simulink model "CLVF"  (R2020a)
settings: Solver=FixedStepAuto  StartTime=0.0  StopTime=tsim  FixedStep=baseRate  RelTol=1e-3  EnableMultiTasking=on
values from neighbouring files (symbols this model uses):
  a = sqrt(sum(aTimesOVec.^2))    [Run_Initializer.m]
  a_max = u_max_scalar/BLACKMass    [Run_Initializer.m]
  a_prime = 0.2    [Run_Initializer.m]
  acceptableRadius = 0.05    [Run_Initializer.m]
  aTimesOVec = d + a_prime*o_hat_prime    [Run_Initializer.m]
  b = 1.0    (= 1)    [Run_Initializer.m]    (also in a_max_CLVF3D_quad.m = params(3))
  baseRate = 0.05    [Run_Initializer.m]
  BLACKInertia = model_param(4)    [Run_Initializer.m]
  BLACKMass = model_param(3)    [Run_Initializer.m]
  cntThreshold = timeThreshold/baseRate    (= 100)    [Run_Initializer.m]
  d = [0.16;0.542;0]    [Run_Initializer.m]
  drop_states_BLACK = rC_I0    [Run_Initializer.m]
  drop_states_BLUE = [ xLength/2+0.9; yLength/2+0.5; 0]    [Run_Initializer.m]
  drop_states_RED = rT_I0    [Run_Initializer.m]
  F_thrusters_BLACK = 0.25.*ones(8,1)    [Run_Initializer.m]
  F_thrusters_BLUE = 0.25.*ones(8,1)    [Run_Initializer.m]
  F_thrusters_RED = 0.25.*ones(8,1)    [Run_Initializer.m]
  finalAngle = fact*pi    (= 2.98451302091)    [Run_Initializer.m]
  home_states_BLACK = [xLength/2-0.4; yLength/2; 0]    [Run_Initializer.m]
  home_states_BLUE = [ xLength/2-0.9; yLength/2+0.5; 0]    [Run_Initializer.m]
  home_states_RED = [xLength/2+0.4; yLength/2; 0]    [Run_Initializer.m]
  init_states_BLACK = rC_I0    [Run_Initializer.m]
  init_states_BLUE = [ xLength/2+0.9; yLength/2+0.5; 0]    [Run_Initializer.m]
  init_states_RED = rT_I0    [Run_Initializer.m]
  ka = 0.01    [Run_Initializer.m]    (also in a_max_CLVF3D_quad.m = params(1))
  kc = 0.01    [Run_Initializer.m]    (also in a_max_CLVF3D_quad.m = params(2))
  kd = 5.0    (= 5)    [Run_Initializer.m]
  Kd_tb = 0.4    [Run_Initializer.m]
  Kd_tblue = 0.4    [Run_Initializer.m]
  Kd_tr = 0.4    [Run_Initializer.m]
  Kd_xb = 5    [Run_Initializer.m]
  Kd_xblue = 5    [Run_Initializer.m]
  Kd_xr = 5    [Run_Initializer.m]
  Kd_yb = 5    [Run_Initializer.m]
  Kd_yblue = 5    [Run_Initializer.m]
  Kd_yr = 5    [Run_Initializer.m]
  Kp_tb = 0.1    [Run_Initializer.m]
  Kp_tblue = 0.1    [Run_Initializer.m]
  Kp_tr = 0.1    [Run_Initializer.m]
  Kp_xb = 2    [Run_Initializer.m]
  Kp_xblue = 2    [Run_Initializer.m]
  Kp_xr = 2    [Run_Initializer.m]
  Kp_yb = 2    [Run_Initializer.m]
  Kp_yblue = 2    [Run_Initializer.m]
  Kp_yr = 2    [Run_Initializer.m]
  MPCStructure = getMPCStructure(BLACKMass, b_cone, R, Q, Q_final, u_max_scalar, kc, aTimesOVec)    [Run_Initializer.m]
  noise_variance_BLACK = 0    [Run_Initializer.m]
  noise_variance_BLUE = 0    [Run_Initializer.m]
  noise_variance_RED = 0    [Run_Initializer.m]
  o_hat_B = aTimesOVec./a    [Run_Initializer.m]
  o_hat_prime = [0;1;0]    [Run_Initializer.m]
  Phase0_End = Phase0_Duration    (= 10)    [Run_Initializer.m]
  Phase1_End = Phase0_Duration + Phase1_Duration    (= 15)    [Run_Initializer.m]
  Phase2_End = Phase0_Duration + Phase1_Duration +                                   Phase2_Duration    (= 35)    [Run_Initializer.m]
  Phase3_End = Phase0_Duration + Phase1_Duration +                                   Phase2_Duration + Phase3_Duration    [Run_Initializer.m]
  Phase3_SubPhase1_End = Phase2_End + Phase3_SubPhase1_Duration    (= 40)    [Run_Initializer.m]
  Phase3_SubPhase2_End = Phase2_End + Phase3_SubPhase1_Duration +                                   Phase3_SubPhase2_Duration    (= 45)    [Run_Initializer.m]
  Phase3_SubPhase3_End_BLACK = Phase2_End + Phase3_SubPhase1_Duration +                                   Phase3_SubPhase2_Duration +                                  Phase3_SubPhase3_Duration + Phase3_SubPhase3_and_a_half    (= 51)    [Run_Initializer.m]
  Phase3_SubPhase3_End_RED = Phase2_End + Phase3_SubPhase1_Duration +                                   Phase3_SubPhase2_Duration +                                  Phase3_SubPhase3_Duration    (= 46)    [Run_Initializer.m]
  Phase3_SubPhase4_End = Phase2_End + Phase3_SubPhase1_Duration +                                   Phase3_SubPhase2_Duration +                                  Phase3_SubPhase3_Duration +                                  Phase3_SubPhase4_Duration + Phase3_SubPhase3_and_a_half    [Run_Initializer.m]
  Phase4_End = Phase0_Duration + Phase1_Duration +                                   Phase2_Duration + Phase3_Duration +                                   Phase4_Duration    [Run_Initializer.m]
  Phase5_End = Phase0_Duration + Phase1_Duration +                                   Phase2_Duration + Phase3_Duration +                                   Phase4_Duration + Phase5_Duration    [Run_Initializer.m]
  rT_I0 = ICStructure.rT_I0{initialConditionSet}    [Run_Initializer.m]
  serverRate = 0.1    [Run_Initializer.m]
  theta_d = 30*d2r    (= 0.523598775598)    [Run_Initializer.m]    (also in a_max_LVF3D.m = rotStuff(4))
  thruster_dist2CG_BLACK = [83.42;-52.58;55.94;-60.05;54.08;-53.92;77.06;-55.94]    [Run_Initializer.m]
  thruster_dist2CG_BLUE = [83.42;-52.58;55.94;-60.05;54.08;-53.92;77.06;-55.94]    [Run_Initializer.m]
  thruster_dist2CG_RED = [49.92;-78.08;70.46;-63.54;81.08;-50.42;57.44;-75.96]    [Run_Initializer.m]
  v_max = interiorPointLVF_heur(     a_prime,      v_max,      a_max,      w_max,      rotNorm,      dockingPortNorm,      theta_d,      fact,      W_LVF,      mu,      tol,      gamma,      beta,      muFact,      muLimit )    [Run_Initializer.m]
  w_body = ICStructure.w_body{initialConditionSet}    [Run_Initializer.m]
undefined symbols (not defined in the file or in its folder): A_cone, DiscIntNeverNeededParam, FixedStep, Phase3_SubPhase3_End, platformSelection, simMode, WhoAmI
libraries: dspstat3 x18, dspsigops x11, raspberrypiBasiclib x10, embdlinuxlib x8, simulink x8, mspfiltlib x3, dsparch4 x3, dspswit3 x2, MainLibrary x2, sensehatlib x1
(part 9 of 10)

== system CLVF/Grab PhaseSpace Data via UDP/Use Hardware to Obtain States/Using RED+BLACK, or RED+BLACK+ARM/Obtain RED States/x_dot -> x2/Hold this value ==
  In1 : Inport
  Action Port : ActionPort  ActionPortLabel=if(u1 ~= 0)
  Out1 : Outport  VectorParamsAs1DForOutWhenUnconnected=off
  wires:
  In1/1 -> Out1/1

== system CLVF/Grab PhaseSpace Data via UDP/Use Hardware to Obtain States/Using RED+BLACK, or RED+BLACK+ARM/Obtain RED States/x_dot -> x3/Hold this value ==
  In1 : Inport
  Action Port : ActionPort  ActionPortLabel=if(u1 ~= 0)
  Out1 : Outport  VectorParamsAs1DForOutWhenUnconnected=off
  wires:
  In1/1 -> Out1/1

== system CLVF/Grab PhaseSpace Data via UDP/Use Hardware to Obtain States/Using RED+BLACK, or RED+BLACK+ARM/Obtain RED States/x_dot -> x4/Hold this value ==
  In1 : Inport
  Action Port : ActionPort  ActionPortLabel=if(u1 ~= 0)
  Out1 : Outport  VectorParamsAs1DForOutWhenUnconnected=off
  wires:
  In1/1 -> Out1/1

== system CLVF/Grab PhaseSpace Data via UDP/Use Hardware to Obtain States/Using RED+BLACK, or RED+BLACK+ARM/Obtain RED States/x_dot -> x5/Hold this value ==
  In1 : Inport
  Action Port : ActionPort  ActionPortLabel=if(u1 ~= 0)
  Out1 : Outport  VectorParamsAs1DForOutWhenUnconnected=off
  wires:
  In1/1 -> Out1/1

== system CLVF/Grab PhaseSpace Data via UDP/Use Hardware to Obtain States/Using RED+BLACK, or RED+BLACK+ARM/Obtain RED States/x_dot -> x6/Hold this value ==
  In1 : Inport
  Action Port : ActionPort  ActionPortLabel=if(u1 ~= 0)
  Out1 : Outport  VectorParamsAs1DForOutWhenUnconnected=off
  wires:
  In1/1 -> Out1/1

== system CLVF/Grab PhaseSpace Data via UDP/Use Hardware to Obtain States/Using RED+BLACK, or RED+BLACK+ARM/Obtain RED States/x_dot -> x7/Hold this value ==
  In1 : Inport
  Action Port : ActionPort  ActionPortLabel=if(u1 ~= 0)
  Out1 : Outport  VectorParamsAs1DForOutWhenUnconnected=off
  wires:
  In1/1 -> Out1/1

== system CLVF/Grab PhaseSpace Data via UDP/Use Hardware to Obtain States/Using RED+BLACK, or RED+BLACK+ARM/Obtain RED States/x_dot -> x8/Hold this value ==
  In1 : Inport
  Action Port : ActionPort  ActionPortLabel=if(u1 ~= 0)
  Out1 : Outport  VectorParamsAs1DForOutWhenUnconnected=off
  wires:
  In1/1 -> Out1/1

== system CLVF/Grab PhaseSpace Data via UDP/Use Hardware to Obtain States/Using RED+BLACK, or RED+BLACK+ARM/Obtain RED States/x_dot -> x9/Hold this value ==
  In1 : Inport
  Action Port : ActionPort  ActionPortLabel=if(u1 ~= 0)
  Out1 : Outport  VectorParamsAs1DForOutWhenUnconnected=off
  wires:
  In1/1 -> Out1/1

== system CLVF/Phase #3: Experiment/Change BLACK Behavior/Sub-Phase #1/Custom Discrete PD (Attitude)/x_dot -> x1/Hold this value ==
  In1 : Inport
  Action Port : ActionPort  ActionPortLabel=if(u1 ~= 0)
  Out1 : Outport  VectorParamsAs1DForOutWhenUnconnected=off
  wires:
  In1/1 -> Out1/1

== system CLVF/Phase #3: Experiment/Change BLACK Behavior/Sub-Phase #1/Custom Discrete PD (X-Position)/x_dot -> x1/Hold this value ==
  In1 : Inport
  Action Port : ActionPort  ActionPortLabel=if(u1 ~= 0)
  Out1 : Outport  VectorParamsAs1DForOutWhenUnconnected=off
  wires:
  In1/1 -> Out1/1

== system CLVF/Phase #3: Experiment/Change BLACK Behavior/Sub-Phase #1/Custom Discrete PD (Y-Position)/x_dot -> x1/Hold this value ==
  In1 : Inport
  Action Port : ActionPort  ActionPortLabel=if(u1 ~= 0)
  Out1 : Outport  VectorParamsAs1DForOutWhenUnconnected=off
  wires:
  In1/1 -> Out1/1

== system CLVF/Phase #3: Experiment/Change BLACK Behavior/Sub-Phase #4/Custom Discrete PD (Attitude)/x_dot -> x1/Hold this value ==
  In1 : Inport
  Action Port : ActionPort  ActionPortLabel=if(u1 ~= 0)
  Out1 : Outport  VectorParamsAs1DForOutWhenUnconnected=off
  wires:
  In1/1 -> Out1/1

== system CLVF/Phase #3: Experiment/Change BLACK Behavior/Sub-Phase #4/Lyapunov GNC/CLVF//LVF System/CLVF ==
  rC_I : Inport
  rT_I : Inport  Port=2
  vT_I : Inport  Port=3
  aT_I : Inport  Port=4
  CT_BI : Inport  Port=5
  wT_B : Inport  Port=6
  w_dot_B : Inport  Port=7
  vC_I : Inport  Port=8
  Action Port : ActionPort  ActionPortLabel=if(u1 == 0)
  Constant : Constant  Value=o_hat_B
  Constant1 : Constant  Value=a
  Constant2 : Constant  Value=b
  Constant3 : Constant  Value=ka
  Constant4 : Constant  Value=kc
  Derivative : Derivative
  Lyapunov Guidance + FF : MATLAB Function  TreatAsAtomicUnit=on
  Scope : Scope
  Scope1 : Scope
  Sum : Sum  Inputs=|+-
  h : Outport
  a_ff : Outport  Port=2
  wires:
  vT_I/1 -> Lyapunov Guidance + FF/3(vT_I)
  rT_I/1 -> Lyapunov Guidance + FF/2(rT_I)
  wT_B/1 -> Lyapunov Guidance + FF/6(wT_B)
  w_dot_B/1 -> Lyapunov Guidance + FF/7(w_dot_B)
  vC_I/1 -> Lyapunov Guidance + FF/8(vC_I)
  CT_BI/1 -> Lyapunov Guidance + FF/5(CT_BI)
  aT_I/1 -> Lyapunov Guidance + FF/4(aT_I)
  rC_I/1 -> Lyapunov Guidance + FF/1(rC_I)
  Lyapunov Guidance + FF/2(a_ff) -> Sum/2, Scope1/1, a_ff/1
  Lyapunov Guidance + FF/1(h) -> Derivative/1, h/1
  Derivative/1 -> Sum/1
  Sum/1 -> Scope/1
  Constant/1 -> Lyapunov Guidance + FF/9(o_hat_B)
  Constant4/1 -> Lyapunov Guidance + FF/13(kc)
  Constant2/1 -> Lyapunov Guidance + FF/11(b)
  Constant3/1 -> Lyapunov Guidance + FF/12(ka)
  Constant1/1 -> Lyapunov Guidance + FF/10(a)

== system CLVF/Phase #3: Experiment/Change BLACK Behavior/Sub-Phase #4/Lyapunov GNC/CLVF//LVF System/Control ==
  h : Inport
  vC_I : Inport  Port=2
  a_ff : Inport  Port=3
  Constant : Constant  Value=m
  Constant1 : Constant  Value=kd
  PD + FF Controller : MATLAB Function  TreatAsAtomicUnit=on
  f : Outport
  wires:
  vC_I/1 -> PD + FF Controller/2(vC_I)
  a_ff/1 -> PD + FF Controller/3(a_ff)
  PD + FF Controller/1(f) -> f/1
  h/1 -> PD + FF Controller/1(h)
  Constant/1 -> PD + FF Controller/4(m)
  Constant1/1 -> PD + FF Controller/5(kd)

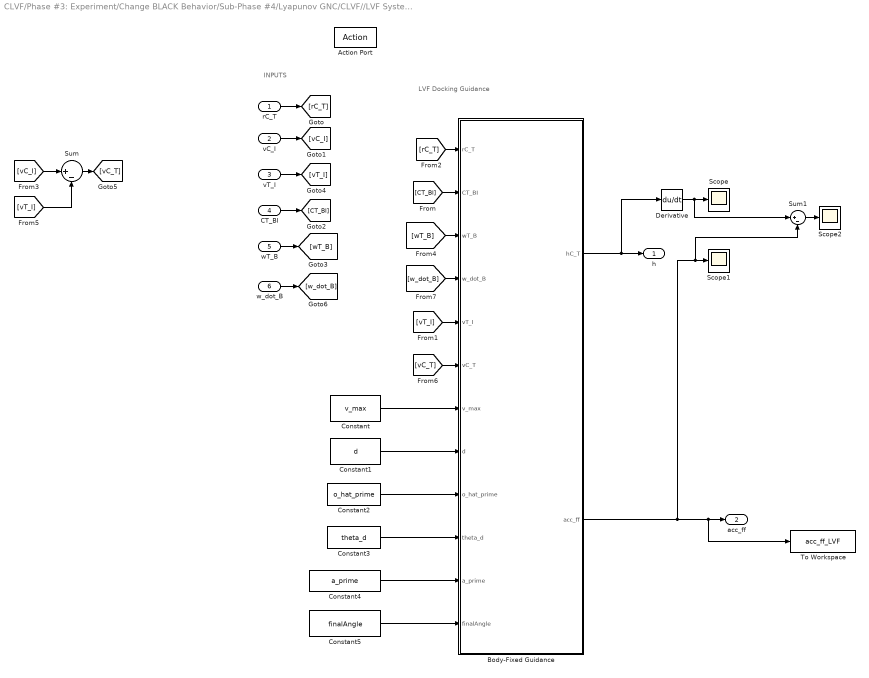
== system CLVF/Phase #3: Experiment/Change BLACK Behavior/Sub-Phase #4/Lyapunov GNC/CLVF//LVF System/Lyapunov ==
  note: LVF Docking Guidance
  note: INPUTS
  rC_T : Inport
  vC_I : Inport  Port=2
  vT_I : Inport  Port=3
  CT_BI : Inport  Port=4
  wT_B : Inport  Port=5
  w_dot_B : Inport  Port=6
  Action Port : ActionPort  ActionPortLabel=else
  Body-Fixed Guidance : MATLAB Function  TreatAsAtomicUnit=on
  Constant : Constant  Value=v_max
  Constant1 : Constant  Value=d
  Constant2 : Constant  Value=o_hat_prime
  Constant3 : Constant  Value=theta_d
  Constant4 : Constant  Value=a_prime
  Constant5 : Constant  Value=finalAngle
  Derivative : Derivative
  Scope : Scope
  Scope1 : Scope
  Scope2 : Scope
  Sum : Sum  Inputs=|+-
  Sum1 : Sum  Inputs=|+-
  To Workspace : ToWorkspace  VariableName=acc_ff_LVF  SampleTime=-1
  h : Outport
  acc_ff : Outport  Port=2
  wires:
  rC_T/1 -> [rC_T]
  vC_I/1 -> [vC_I]
  CT_BI/1 -> [CT_BI]
  wT_B/1 -> [wT_B]
  [rC_T] -> Body-Fixed Guidance/1(rC_T)
  [wT_B] -> Body-Fixed Guidance/3(wT_B)
  [CT_BI] -> Body-Fixed Guidance/2(CT_BI)
  [w_dot_B] -> Body-Fixed Guidance/4(w_dot_B)
  vT_I/1 -> [vT_I]
  Body-Fixed Guidance/1(hC_T) -> Derivative/1, h/1
  [vT_I] -> Body-Fixed Guidance/5(vT_I)
  [vC_I] -> Sum/1
  [vT_I] -> Sum/2
  Sum/1 -> [vC_T]
  [vC_T] -> Body-Fixed Guidance/6(vC_T)
  Body-Fixed Guidance/2(acc_ff) -> Sum1/2, Scope1/1, To Workspace/1, acc_ff/1
  Derivative/1 -> Sum1/1, Scope/1
  Sum1/1 -> Scope2/1
  w_dot_B/1 -> [w_dot_B]
  Constant/1 -> Body-Fixed Guidance/7(v_max)
  Constant1/1 -> Body-Fixed Guidance/8(d)
  Constant2/1 -> Body-Fixed Guidance/9(o_hat_prime)
  Constant3/1 -> Body-Fixed Guidance/10(theta_d)
  Constant4/1 -> Body-Fixed Guidance/11(a_prime)
  Constant5/1 -> Body-Fixed Guidance/12(finalAngle)

== system CLVF/Phase #3: Experiment/Change BLACK Behavior/Sub-Phase #4/Lyapunov GNC/CLVF//LVF System/SWITCH ==
  rC_T : Inport
  C_BI : Inport  Port=2
  Constant : Constant  Value=aTimesOVec
  Constant1 : Constant  Value=acceptableDistance
  Constant2 : Constant  Value=cntThreshold
  Delay : Delay  DelayLength=1  InitialCondition=0
  Sample and Hold : dspsigops/Sample and Hold  trig=Rising edge  initCond=0  latchinput=off
  inDesiredRadius : MATLAB Function  TreatAsAtomicUnit=on
  sufficientTime : MATLAB Function  TreatAsAtomicUnit=on
  oneOrZero : Outport
  wires:
  rC_T/1 -> inDesiredRadius/1(rC_T)
  Delay/1 -> inDesiredRadius/2(currentCnt)
  inDesiredRadius/1(newCnt) -> sufficientTime/1(cnt), Delay/1
  Sample and Hold/1 -> oneOrZero/1
  sufficientTime/1(oneOrZero) -> Sample and Hold/1, Sample and Hold/Trigger
  Constant1/1 -> inDesiredRadius/3(acceptableDistance)
  Constant2/1 -> sufficientTime/2(cntThreshold)
  C_BI/1 -> inDesiredRadius/4(C_BI)
  Constant/1 -> inDesiredRadius/5(aTimesOVec)

== system CLVF/Phase #3: Experiment/Change BLACK Behavior/Sub-Phase #4/Lyapunov GNC/Navigation/Vec Derivative ==
  In1 : Inport
  Demux4 : Demux  Outputs=3
  Mux : Mux  Inputs=3
  "x_dot -> x1" : Subsystem
  "x_dot -> x2" : Subsystem
  "x_dot -> x3" : Subsystem
  vC_I : Outport  VectorParamsAs1DForOutWhenUnconnected=off
  wires:
  Demux4/1 -> "x_dot -> x1"/1(y(t))
  Demux4/2 -> "x_dot -> x2"/1(y(t))
  Demux4/3 -> "x_dot -> x3"/1(y(t))
  "x_dot -> x2"/1(dy(t)/dt) -> Mux/2
  In1/1 -> Demux4/1
  Mux/1 -> vC_I/1
  "x_dot -> x1"/1(dy(t)/dt) -> Mux/1
  "x_dot -> x3"/1(dy(t)/dt) -> Mux/3

== system CLVF/Phase #3: Experiment/Change BLACK Behavior/Sub-Phase #4/Lyapunov GNC/Navigation/x_dot -> x3 ==
  note: dy/dt ~= (y2-y1)/deltaT
  y(t) : Inport
  Delay1 : Delay  DelayLength=1  InitialConditionSource=Input port
      settings: InputPortMap=u0,p4
  Hold this value : Subsystem  TreatAsAtomicUnit=on
  Sum6 : Sum  Inputs=-+|
  divide by delta T : Gain  Gain=1/serverRate
  "if we went through a \"step\"" : If  IfExpression=u1 ~= 0  ShowElse=off
  dy(t)/dt : Outport  VectorParamsAs1DForOutWhenUnconnected=off
  wires:
  divide by delta T/1 -> dy(t)/dt/1
  Delay1/1 -> Sum6/1
  "if we went through a \"step\""/1 -> Hold this value/Action
  Hold this value/1(Out1) -> divide by delta T/1
  Sum6/1 -> "if we went through a \"step\""/1, Hold this value/1(In1)
  y(t)/1 -> Sum6/2, Delay1/2, Delay1/1

== system CLVF/Phase #3: Experiment/Change BLACK Behavior/Sub-Phase #4/Lyapunov GNC/Subsystem/Inner MPC ==
  x_mes : Inport
  target_angles_mes : Inport  Port=2
  mes_ang_vel : Inport  Port=3
  Action Port : ActionPort  PropagateVarSize=During execution  ActionPortLabel=else
  Constant : Constant
  Inner MPC : Subsystem  SystemSampleTime=FixedStep  mask{t_vec=MPCStructure.future_time_vector, J_z=BLACKInertia, J_transverse=0, u_con_mat=MPCStructure.u_con_mat, u_con_vec=MPCStructure.u_con_vec, x_con_mat_0=MPCStructure.x_con_mat, x_con_vec=MPCStructure.x_con_vec, Np=MPCStructure.Np, d=d, A_cone=A_cone, Q=MPCStructure.Q, Aeq=MPCStructure.Aeq, warm_start_matrix=MPCStructure.warm_start_matrix, A_discrete=MPCStructure.A_d, K_feedback=0, X0=MPCStructure.X0, beq_size=MPCStructure.N_INEQ_INNER, LB=MPCStructure.LB, UB=MPCStructure.UB, N_INEQ_INNER=MPCStructure.N_INEQ_INNER, N_EQ=MPCStructure.N_EQ, X_SIZE=MPCStructure.X_SIZE}
      mask prompts: t_vec "future time vector"; J_z "Inertia (sym axis)"; J_transverse "Inertia (trans axis)"; u_con_mat "u constraint matrix"; u_con_vec "u constraint vector"; x_con_mat_0 "x constraint matrix (proper size at least)"; x_con_vec "x constraint vector"; Np "Time horizon in steps"; d "Docking port in body-frame"; A_cone "Cone constraint matrix"; Q "Cost Matrix"; Aeq "Equality constraint matrix"; warm_start_matrix "warm start matrix"; A_discrete "A matrix (discrete system)"; K_feedback "Feedback Gain"; X0 "Initial optimizer guess"; beq_size "Height of equality matrix"; LB "Lower Bound Vector"; UB "Upper Bound Vector"; N_INEQ_INNER "Number of inequality constrain"; N_EQ "Number of equality const"; X_SIZE "Size of X vector"
      mask help: This block runs a docking MPC controller for a axi-symmetric target spacecraft.
  u : Outport
  zone : Outport  Port=2
  wires:
  Inner MPC/1(u) -> u/1
  x_mes/1 -> Inner MPC/1(x_mes)
  target_angles_mes/1 -> Inner MPC/2(theta_T)
  mes_ang_vel/1 -> Inner MPC/3(theta_dot_T)
  Constant/1 -> zone/1

== system CLVF/Phase #3: Experiment/Change BLACK Behavior/Sub-Phase #4/Lyapunov GNC/Subsystem/Outer MPC ==
  x_mes : Inport
  mes_theta : Inport  Port=2
  mes_theta_dot : Inport  Port=3
  Action Port : ActionPort  PropagateVarSize=During execution  ActionPortLabel=if(u1 == 0)
  Constant : Constant  Value=0
  Outer MPC : Subsystem  SystemSampleTime=FixedStep  mask{t_vec=MPCStructure.future_time_vector, J_z=BLACKInertia, J_transverse=0, Np=MPCStructure.Np, Q=MPCStructure.Q, Aeq=MPCStructure.Aeq, warm_start_matrix=MPCStructure.warm_start_matrix, A_discrete=MPCStructure.A_d, K_feedback=0, X0=MPCStructure.X0, beq_size=MPCStructure.N_INEQ_OUTER, LB=MPCStructure.LB, UB=MPCStructure.UB, tracking_point=MPCStructure.tracking_point, r_safe=a, X_SIZE=MPCStructure.X_SIZE, N_INEQ_OUTER=MPCStructure.N_INEQ_OUTER, N_EQ=MPCStructure.N_EQ}
      mask prompts: t_vec "future time vector"; J_z "Inertia (sym axis)"; J_transverse "Inertia (trans axis)"; Np "Time horizon in steps"; Q "Cost Matrix"; Aeq "Equality constraint matrix"; warm_start_matrix "warm start matrix"; A_discrete "A matrix (discrete system)"; K_feedback "Feedback Gain"; X0 "Initial optimizer guess"; beq_size "Height of equality matrix"; LB "Lower Bound Vector"; UB "Upper Bound Vector"; tracking_point "Tracking Point"; r_safe "Safe distance around target"; X_SIZE "Size of X vector"; N_INEQ_OUTER "Number of inequality constr."; N_EQ "Number of equality constr."
      mask help: This block runs a docking MPC controller for a axi-symmetric target spacecraft.
  u : Outport
  zone : Outport  Port=2
  wires:
  Outer MPC/1(u) -> u/1
  x_mes/1 -> Outer MPC/1(x_mes)
  mes_theta/1 -> Outer MPC/2(mes_theta)
  mes_theta_dot/1 -> Outer MPC/3(mes_theta_dot)
  Constant/1 -> zone/1

== system CLVF/Phase #3: Experiment/Change BLACK Behavior/Sub-Phase #4/Lyapunov GNC/Subsystem/SWITCH ==
  rC_T : Inport
  C_BI : Inport  Port=2
  Constant : Constant  Value=aTimesOVec
  Constant1 : Constant  Value=acceptableRadius
  Constant2 : Constant  Value=cntThreshold
  Delay : Delay  DelayLength=1  InitialCondition=0
  Sample and Hold : dspsigops/Sample and Hold  trig=Rising edge  initCond=0  latchinput=off
  inDesiredRadius : MATLAB Function  TreatAsAtomicUnit=on
  sufficientTime : MATLAB Function  TreatAsAtomicUnit=on
  oneOrZero : Outport
  wires:
  rC_T/1 -> inDesiredRadius/1(rC_T)
  Delay/1 -> inDesiredRadius/2(currentCnt)
  inDesiredRadius/1(newCnt) -> sufficientTime/1(cnt), Delay/1
  Sample and Hold/1 -> oneOrZero/1
  sufficientTime/1(oneOrZero) -> Sample and Hold/1, Sample and Hold/Trigger
  Constant1/1 -> inDesiredRadius/3(acceptableDistance)
  Constant2/1 -> sufficientTime/2(cntThreshold)
  C_BI/1 -> inDesiredRadius/4(C_BI)
  Constant/1 -> inDesiredRadius/5(aTimesOVec)

== system CLVF/Phase #3: Experiment/Change BLUE Behavior/Sub-Phase #1/Custom Discrete PD (Attitude)/x_dot -> x1/Hold this value ==
  In1 : Inport
  Action Port : ActionPort  ActionPortLabel=if(u1 ~= 0)
  Out1 : Outport  VectorParamsAs1DForOutWhenUnconnected=off
  wires:
  In1/1 -> Out1/1

== system CLVF/Phase #3: Experiment/Change BLUE Behavior/Sub-Phase #1/Custom Discrete PD (X-Position)/x_dot -> x1/Hold this value ==
  In1 : Inport
  Action Port : ActionPort  ActionPortLabel=if(u1 ~= 0)
  Out1 : Outport  VectorParamsAs1DForOutWhenUnconnected=off
  wires:
  In1/1 -> Out1/1

== system CLVF/Phase #3: Experiment/Change BLUE Behavior/Sub-Phase #1/Custom Discrete PD (Y-Position)/x_dot -> x1/Hold this value ==
  In1 : Inport
  Action Port : ActionPort  ActionPortLabel=if(u1 ~= 0)
  Out1 : Outport  VectorParamsAs1DForOutWhenUnconnected=off
  wires:
  In1/1 -> Out1/1

== system CLVF/Phase #3: Experiment/Change BLUE Behavior/Sub-Phase #4/Custom Discrete PD (Attitude)/x_dot -> x1/Hold this value ==
  In1 : Inport
  Action Port : ActionPort  ActionPortLabel=if(u1 ~= 0)
  Out1 : Outport  VectorParamsAs1DForOutWhenUnconnected=off
  wires:
  In1/1 -> Out1/1

== system CLVF/Phase #3: Experiment/Change BLUE Behavior/Sub-Phase #4/Custom Discrete PD (X-Position)/x_dot -> x1/Hold this value ==
  In1 : Inport
  Action Port : ActionPort  ActionPortLabel=if(u1 ~= 0)
  Out1 : Outport  VectorParamsAs1DForOutWhenUnconnected=off
  wires:
  In1/1 -> Out1/1

== system CLVF/Phase #3: Experiment/Change BLUE Behavior/Sub-Phase #4/Custom Discrete PD (Y-Position)/x_dot -> x1/Hold this value ==
  In1 : Inport
  Action Port : ActionPort  ActionPortLabel=if(u1 ~= 0)
  Out1 : Outport  VectorParamsAs1DForOutWhenUnconnected=off
  wires:
  In1/1 -> Out1/1

== system CLVF/Phase #3: Experiment/Change RED Behavior/Sub-Phase #1/Custom Discrete PD (Attitude)/x_dot -> x1/Hold this value ==
  In1 : Inport
  Action Port : ActionPort  ActionPortLabel=if(u1 ~= 0)
  Out1 : Outport  VectorParamsAs1DForOutWhenUnconnected=off
  wires:
  In1/1 -> Out1/1

== system CLVF/Phase #3: Experiment/Change RED Behavior/Sub-Phase #1/Custom Discrete PD (X-Position)/x_dot -> x1/Hold this value ==
  In1 : Inport
  Action Port : ActionPort  ActionPortLabel=if(u1 ~= 0)
  Out1 : Outport  VectorParamsAs1DForOutWhenUnconnected=off
  wires:
  In1/1 -> Out1/1

== system CLVF/Phase #3: Experiment/Change RED Behavior/Sub-Phase #1/Custom Discrete PD (Y-Position)/x_dot -> x1/Hold this value ==
  In1 : Inport
  Action Port : ActionPort  ActionPortLabel=if(u1 ~= 0)
  Out1 : Outport  VectorParamsAs1DForOutWhenUnconnected=off
  wires:
  In1/1 -> Out1/1

== system CLVF/Phase #3: Experiment/Change RED Behavior/Sub-Phase #4/Custom Discrete PD (Attitude)/x_dot -> x1/Hold this value ==
  In1 : Inport
  Action Port : ActionPort  ActionPortLabel=if(u1 ~= 0)
  Out1 : Outport  VectorParamsAs1DForOutWhenUnconnected=off
  wires:
  In1/1 -> Out1/1

== system CLVF/Phase #3: Experiment/Change RED Behavior/Sub-Phase #4/Custom Discrete PD (X-Position)/x_dot -> x1/Hold this value ==
  In1 : Inport
  Action Port : ActionPort  ActionPortLabel=if(u1 ~= 0)
  Out1 : Outport  VectorParamsAs1DForOutWhenUnconnected=off
  wires:
  In1/1 -> Out1/1

== system CLVF/Phase #3: Experiment/Change RED Behavior/Sub-Phase #4/Custom Discrete PD (Y-Position)/x_dot -> x1/Hold this value ==
  In1 : Inport
  Action Port : ActionPort  ActionPortLabel=if(u1 ~= 0)
  Out1 : Outport  VectorParamsAs1DForOutWhenUnconnected=off
  wires:
  In1/1 -> Out1/1

== system CLVF/Phase #3: Experiment/Change BLACK Behavior/Sub-Phase #4/Lyapunov GNC/Navigation/Vec Derivative/x_dot -> x1 ==
  note: dy/dt ~= (y2-y1)/deltaT
  y(t) : Inport
  Delay1 : Delay  DelayLength=1  InitialConditionSource=Input port
      settings: InputPortMap=u0,p4
  Hold this value : Subsystem  TreatAsAtomicUnit=on
  Sum6 : Sum  Inputs=-+|
  divide by delta T : Gain  Gain=1/serverRate
  "if we went through a \"step\"" : If  IfExpression=u1 ~= 0  ShowElse=off
  dy(t)/dt : Outport  VectorParamsAs1DForOutWhenUnconnected=off
  wires:
  divide by delta T/1 -> dy(t)/dt/1
  Delay1/1 -> Sum6/1
  "if we went through a \"step\""/1 -> Hold this value/Action
  Hold this value/1(Out1) -> divide by delta T/1
  Sum6/1 -> "if we went through a \"step\""/1, Hold this value/1(In1)
  y(t)/1 -> Sum6/2, Delay1/2, Delay1/1

== system CLVF/Phase #3: Experiment/Change BLACK Behavior/Sub-Phase #4/Lyapunov GNC/Navigation/Vec Derivative/x_dot -> x2 ==
  note: dy/dt ~= (y2-y1)/deltaT
  y(t) : Inport
  Delay1 : Delay  DelayLength=1  InitialConditionSource=Input port
      settings: InputPortMap=u0,p4
  Hold this value : Subsystem  TreatAsAtomicUnit=on
  Sum6 : Sum  Inputs=-+|
  divide by delta T : Gain  Gain=1/serverRate
  "if we went through a \"step\"" : If  IfExpression=u1 ~= 0  ShowElse=off
  dy(t)/dt : Outport  VectorParamsAs1DForOutWhenUnconnected=off
  wires:
  divide by delta T/1 -> dy(t)/dt/1
  Delay1/1 -> Sum6/1
  "if we went through a \"step\""/1 -> Hold this value/Action
  Hold this value/1(Out1) -> divide by delta T/1
  Sum6/1 -> "if we went through a \"step\""/1, Hold this value/1(In1)
  y(t)/1 -> Sum6/2, Delay1/2, Delay1/1

== system CLVF/Phase #3: Experiment/Change BLACK Behavior/Sub-Phase #4/Lyapunov GNC/Navigation/Vec Derivative/x_dot -> x3 ==
  note: dy/dt ~= (y2-y1)/deltaT
  y(t) : Inport
  Delay1 : Delay  DelayLength=1  InitialConditionSource=Input port
      settings: InputPortMap=u0,p4
  Hold this value : Subsystem  TreatAsAtomicUnit=on
  Sum6 : Sum  Inputs=-+|
  divide by delta T : Gain  Gain=1/serverRate
  "if we went through a \"step\"" : If  IfExpression=u1 ~= 0  ShowElse=off
  dy(t)/dt : Outport  VectorParamsAs1DForOutWhenUnconnected=off
  wires:
  divide by delta T/1 -> dy(t)/dt/1
  Delay1/1 -> Sum6/1
  "if we went through a \"step\""/1 -> Hold this value/Action
  Hold this value/1(Out1) -> divide by delta T/1
  Sum6/1 -> "if we went through a \"step\""/1, Hold this value/1(In1)
  y(t)/1 -> Sum6/2, Delay1/2, Delay1/1

== system CLVF/Phase #3: Experiment/Change BLACK Behavior/Sub-Phase #4/Lyapunov GNC/Navigation/x_dot -> x3/Hold this value ==
  In1 : Inport
  Action Port : ActionPort  ActionPortLabel=if(u1 ~= 0)
  Out1 : Outport  VectorParamsAs1DForOutWhenUnconnected=off
  wires:
  In1/1 -> Out1/1

== system CLVF/Phase #3: Experiment/Change BLACK Behavior/Sub-Phase #4/Lyapunov GNC/Subsystem/Inner MPC/Inner MPC ==
  x_mes : Inport
  theta_T : Inport  Port=2
  theta_dot_T : Inport  Port=3
  Subsystem : Subsystem
  Sum : Sum  Inputs=|++
  "future -> inequality constraints" : Subsystem
  get equality constraint vector : Subsystem
  u_feedback : Subsystem  Commented=on
  u_feedforward MPC : Subsystem
  u : Outport
  wires:
  u_feedforward MPC/1(u_MPC) -> Sum/1
  Sum/1 -> u/1
  x_mes/1 -> get equality constraint vector/1(x0), u_feedback/2(x_est)
  u_feedforward MPC/2(x_next) -> u_feedback/1(x_nom)
  u_feedback/1(u_feedback) -> Sum/2
  "future -> inequality constraints"/1(A) -> u_feedforward MPC/1(A)
  "future -> inequality constraints"/2(b) -> u_feedforward MPC/2(b)
  Subsystem/1(C_BI_Np) -> "future -> inequality constraints"/1(C_BI_Np)
  theta_T/1 -> Subsystem/1(theta_T)
  theta_dot_T/1 -> Subsystem/2(theta_dot_T)
  Subsystem/2(x_des_future) -> u_feedforward MPC/3(x_des_future)
  get equality constraint vector/1(beq) -> u_feedforward MPC/4(beq)

== system CLVF/Phase #3: Experiment/Change BLACK Behavior/Sub-Phase #4/Lyapunov GNC/Subsystem/Outer MPC/Outer MPC ==
  x_mes : Inport
  mes_theta : Inport  Port=2
  mes_theta_dot : Inport  Port=3
  Constant : Constant  Value=tracking_point
  Selector : Selector  InputPortWidth=6  IndexOptions=Index vector (dialog)  Indices=[1:3]  OutputSizes=1
  Subsystem : Subsystem
  Sum : Sum  Inputs=|++
  Terminator : Terminator
  "current position -> inequality constraints" : Subsystem
  get equality constraint vector : Subsystem
  u_feedback : Subsystem  Commented=on
  u_feedforward MPC : Subsystem
  u : Outport
  wires:
  u_feedforward MPC/1(u_MPC) -> Sum/1
  Sum/1 -> u/1
  x_mes/1 -> Selector/1, get equality constraint vector/1(x0), u_feedback/2(x_est)
  u_feedforward MPC/2(x_next) -> u_feedback/1(x_nom)
  u_feedback/1(u_feedback) -> Sum/2
  "current position -> inequality constraints"/1(A) -> u_feedforward MPC/1(A)
  "current position -> inequality constraints"/2(b) -> u_feedforward MPC/2(b)
  mes_theta/1 -> Subsystem/1(mes_theta)
  mes_theta_dot/1 -> Subsystem/2(theta_dot)
  Subsystem/2(x_des_future) -> u_feedforward MPC/3(x_des_future)
  get equality constraint vector/1(beq) -> u_feedforward MPC/4(beq)
  Subsystem/1(C_BI_Np) -> Terminator/1
  Constant/1 -> Subsystem/3(tracking_point)
  Selector/1 -> "current position -> inequality constraints"/1(r0)

== system CLVF/Phase #3: Experiment/Change BLACK Behavior/Sub-Phase #4/Lyapunov GNC/Navigation/Vec Derivative/x_dot -> x1/Hold this value ==
  In1 : Inport
  Action Port : ActionPort  ActionPortLabel=if(u1 ~= 0)
  Out1 : Outport  VectorParamsAs1DForOutWhenUnconnected=off
  wires:
  In1/1 -> Out1/1

== system CLVF/Phase #3: Experiment/Change BLACK Behavior/Sub-Phase #4/Lyapunov GNC/Navigation/Vec Derivative/x_dot -> x2/Hold this value ==
  In1 : Inport
  Action Port : ActionPort  ActionPortLabel=if(u1 ~= 0)
  Out1 : Outport  VectorParamsAs1DForOutWhenUnconnected=off
  wires:
  In1/1 -> Out1/1

== system CLVF/Phase #3: Experiment/Change BLACK Behavior/Sub-Phase #4/Lyapunov GNC/Navigation/Vec Derivative/x_dot -> x3/Hold this value ==
  In1 : Inport
  Action Port : ActionPort  ActionPortLabel=if(u1 ~= 0)
  Out1 : Outport  VectorParamsAs1DForOutWhenUnconnected=off
  wires:
  In1/1 -> Out1/1

== system CLVF/Phase #3: Experiment/Change BLACK Behavior/Sub-Phase #4/Lyapunov GNC/Subsystem/Inner MPC/Inner MPC/Subsystem ==
  theta_T : Inport
  theta_dot_T : Inport  Port=2
  Constant : Constant  Value=t_vec
  Constant3 : Constant  Value=d
  MATLAB Function1 : MATLAB Function  TreatAsAtomicUnit=on
  C_BI_Np : Outport
  x_des_future : Outport  Port=2
  wires:
  Constant/1 -> MATLAB Function1/2(t_vec)
  theta_T/1 -> MATLAB Function1/1(theta_0)
  theta_dot_T/1 -> MATLAB Function1/3(omega_z)
  Constant3/1 -> MATLAB Function1/4(d)
  MATLAB Function1/1(C_BI_Np) -> C_BI_Np/1
  MATLAB Function1/2(x_des_future) -> x_des_future/1

== system CLVF/Phase #3: Experiment/Change BLACK Behavior/Sub-Phase #4/Lyapunov GNC/Subsystem/Inner MPC/Inner MPC/future -> inequality constraints ==
  C_BI_Np : Inport
  Constant : Constant  Value=zeros(N_INEQ_INNER, X_SIZE)
  Constant1 : Constant  Value=zeros(N_INEQ_INNER,1)
  Constant2 : Constant  Value=x_con_mat_0
  Constant3 : Constant  Value=x_con_vec
  Constant4 : Constant  Value=Np
  Constant6 : Constant  Value=A_cone
  Delay : Delay  DelayLength=1  InitialConditionSource=Input port
      settings: InputPortMap=u0,p4
  Delay1 : Delay  DelayLength=1  InitialConditionSource=Input port
      settings: InputPortMap=u0,p4
  MATLAB Function : MATLAB Function  TreatAsAtomicUnit=on
  A : Outport
  b : Outport  Port=2
  wires:
  MATLAB Function/1(A) -> Delay/1, A/1
  C_BI_Np/1 -> MATLAB Function/4(C_BI_Np)
  Constant2/1 -> MATLAB Function/1(x_con_mat)
  Constant3/1 -> MATLAB Function/2(x_con_vec)
  Constant4/1 -> MATLAB Function/3(Np)
  Constant6/1 -> MATLAB Function/5(A_cone)
  MATLAB Function/2(b) -> Delay1/1, b/1
  Delay/1 -> MATLAB Function/6(prev_A)
  Delay1/1 -> MATLAB Function/7(prev_b)
  Constant/1 -> Delay/2
  Constant1/1 -> Delay1/2

== system CLVF/Phase #3: Experiment/Change BLACK Behavior/Sub-Phase #4/Lyapunov GNC/Subsystem/Inner MPC/Inner MPC/get equality constraint vector ==
  x0 : Inport
  Constant : Constant  Value=Np
  Constant1 : Constant  Value=A_discrete
  Constant2 : Constant  Value=zeros(N_EQ, 1)
  Delay : Delay  DelayLength=1  InitialConditionSource=Input port
      settings: InputPortMap=u0,p4
  Gain : Gain  Gain=-1
  MATLAB Function : MATLAB Function  TreatAsAtomicUnit=on
  beq : Outport
  wires:
  x0/1 -> MATLAB Function/3(x0)
  Constant/1 -> MATLAB Function/2(Np)
  Constant1/1 -> MATLAB Function/1(A)
  MATLAB Function/1(p) -> Gain/1
  Gain/1 -> Delay/1, beq/1
  Delay/1 -> MATLAB Function/4(prev_b)
  Constant2/1 -> Delay/2

== system CLVF/Phase #3: Experiment/Change BLACK Behavior/Sub-Phase #4/Lyapunov GNC/Subsystem/Inner MPC/Inner MPC/u_feedback ==
  x_nom : Inport
  x_est : Inport  Port=2
  Constant : Constant  Value=K_feedback
  Matrix Multiply : Product  Multiplication=Matrix(*)
  Sum : Sum  Inputs=|+-
  u_feedback : Outport
  wires:
  x_nom/1 -> Sum/1
  x_est/1 -> Sum/2
  Sum/1 -> Matrix Multiply/2
  Constant/1 -> Matrix Multiply/1
  Matrix Multiply/1 -> u_feedback/1

== system CLVF/Phase #3: Experiment/Change BLACK Behavior/Sub-Phase #4/Lyapunov GNC/Subsystem/Inner MPC/Inner MPC/u_feedforward MPC ==
  A : Inport
  b : Inport  Port=2
  x_des_future : Inport  Port=3
  beq : Inport  Port=4
  Aeq : Constant  Value=Aeq
  Constant : Constant  Value=Q
  Constant1 : Constant  Value=warm_start_matrix
  Constant2 : Constant  Value=X0
  Constant3 : Constant  Value=LB
  Constant4 : Constant  Value=UB
  Delay : Delay  DelayLength=1  InitialConditionSource=Input port
      settings: InputPortMap=u0,p4
  Matrix Multiply : Product  Multiplication=Matrix(*)
  Solve MPC : MATLAB Function  TreatAsAtomicUnit=on
  u_MPC : Outport
  x_next : Outport  Port=2
  wires:
  A/1 -> Solve MPC/2(A)
  Matrix Multiply/1 -> Solve MPC/8(X0)
  beq/1 -> Solve MPC/5(beq)
  Constant1/1 -> Matrix Multiply/1
  Constant/1 -> Solve MPC/1(Q)
  Delay/1 -> Matrix Multiply/2
  Aeq/1 -> Solve MPC/4(Aeq)
  b/1 -> Solve MPC/3(b)
  Solve MPC/3(X) -> Delay/1
  Solve MPC/1(u) -> u_MPC/1
  Solve MPC/2(x_next) -> x_next/1
  x_des_future/1 -> Solve MPC/9(x_des_future)
  Constant2/1 -> Delay/2
  Constant3/1 -> Solve MPC/6(LB)
  Constant4/1 -> Solve MPC/7(UB)

== system CLVF/Phase #3: Experiment/Change BLACK Behavior/Sub-Phase #4/Lyapunov GNC/Subsystem/Outer MPC/Outer MPC/Subsystem ==
  mes_theta : Inport
  theta_dot : Inport  Port=2
  tracking_point : Inport  Port=3
  Constant : Constant  Value=t_vec
  MATLAB Function : MATLAB Function  TreatAsAtomicUnit=on
  C_BI_Np : Outport
  x_des_future : Outport  Port=2
  wires:
  MATLAB Function/1(C_BI_Np) -> C_BI_Np/1
  MATLAB Function/2(x_des_future) -> x_des_future/1
  Constant/1 -> MATLAB Function/2(t_vec)
  mes_theta/1 -> MATLAB Function/1(theta_0)
  theta_dot/1 -> MATLAB Function/3(omega_z)
  tracking_point/1 -> MATLAB Function/4(d)

== system CLVF/Phase #3: Experiment/Change BLACK Behavior/Sub-Phase #4/Lyapunov GNC/Subsystem/Outer MPC/Outer MPC/current position -> inequality constraints ==
  r0 : Inport
  Constant : Constant  Value=N_INEQ_OUTER
  Constant1 : Constant  Value=Np
  Constant2 : Constant  Value=X_SIZE
  Constant8 : Constant  Value=r_safe
  Delay : Delay  DelayLength=1  InitialCondition=zeros(MPCStructure.N_INEQ_OUTER,MPCStructure.X_SIZE)
  Delay1 : Delay  DelayLength=1  InitialCondition=zeros(MPCStructure.N_INEQ_OUTER,1)
  MATLAB Function1 : MATLAB Function  TreatAsAtomicUnit=on
  A : Outport
  b : Outport  Port=2
  wires:
  Constant1/1 -> MATLAB Function1/3(Np)
  Constant8/1 -> MATLAB Function1/2(r_safe)
  r0/1 -> MATLAB Function1/1(r0)
  MATLAB Function1/2(b) -> Delay1/1, b/1
  Delay/1 -> MATLAB Function1/4(prev_A)
  Delay1/1 -> MATLAB Function1/5(prev_b)
  MATLAB Function1/1(A) -> A/1, Delay/1
  Constant/1 -> MATLAB Function1/6(N_INEQ_OUTER)
  Constant2/1 -> MATLAB Function1/7(X_SIZE)

== system CLVF/Phase #3: Experiment/Change BLACK Behavior/Sub-Phase #4/Lyapunov GNC/Subsystem/Outer MPC/Outer MPC/get equality constraint vector ==
  x0 : Inport
  Constant : Constant  Value=Np
  Constant1 : Constant  Value=A_discrete
  Delay : Delay  DelayLength=1  InitialCondition=zeros(MPCStructure.N_EQ,1)
  Gain : Gain  Gain=-1
  MATLAB Function : MATLAB Function  TreatAsAtomicUnit=on
  beq : Outport
  wires:
  x0/1 -> MATLAB Function/3(x0)
  Constant/1 -> MATLAB Function/2(Np)
  Constant1/1 -> MATLAB Function/1(A)
  MATLAB Function/1(p) -> Gain/1, Delay/1
  Delay/1 -> MATLAB Function/4(prev_p)
  Gain/1 -> beq/1

== system CLVF/Phase #3: Experiment/Change BLACK Behavior/Sub-Phase #4/Lyapunov GNC/Subsystem/Outer MPC/Outer MPC/u_feedback ==
  x_nom : Inport
  x_est : Inport  Port=2
  Constant : Constant  Value=K_feedback
  Matrix Multiply : Product  Multiplication=Matrix(*)
  Sum : Sum  Inputs=|+-
  u_feedback : Outport
  wires:
  x_nom/1 -> Sum/1
  x_est/1 -> Sum/2
  Sum/1 -> Matrix Multiply/2
  Constant/1 -> Matrix Multiply/1
  Matrix Multiply/1 -> u_feedback/1

== system CLVF/Phase #3: Experiment/Change BLACK Behavior/Sub-Phase #4/Lyapunov GNC/Subsystem/Outer MPC/Outer MPC/u_feedforward MPC ==
  A : Inport
  b : Inport  Port=2
  x_des_future : Inport  Port=3
  beq : Inport  Port=4
  Aeq : Constant  Value=Aeq
  Constant : Constant  Value=Q
  Constant1 : Constant  Value=warm_start_matrix
  Constant2 : Constant  Value=X0
  Constant3 : Constant  Value=LB
  Constant4 : Constant  Value=UB
  Delay : Delay  DelayLength=1  InitialConditionSource=Input port
      settings: InputPortMap=u0,p4
  Matrix Multiply : Product  Multiplication=Matrix(*)
  Solve MPC : MATLAB Function  TreatAsAtomicUnit=on
  u_MPC : Outport
  x_next : Outport  Port=2
  wires:
  Constant1/1 -> Matrix Multiply/1
  Delay/1 -> Matrix Multiply/2
  Solve MPC/3(X) -> Delay/1
  Constant2/1 -> Delay/2
  Constant/1 -> Solve MPC/1(Q)
  Constant3/1 -> Solve MPC/6(LB)
  Constant4/1 -> Solve MPC/7(UB)
  A/1 -> Solve MPC/2(A)
  b/1 -> Solve MPC/3(b)
  Aeq/1 -> Solve MPC/4(Aeq)
  beq/1 -> Solve MPC/5(beq)
  x_des_future/1 -> Solve MPC/9(x_des_future)
  Solve MPC/1(u) -> u_MPC/1
  Solve MPC/2(x_next) -> x_next/1
  Matrix Multiply/1 -> Solve MPC/8(X0)

== matlab function CLVF/Phase #2: Move to Initial Position/Change BLACK Behavior/Hough Control/MATLAB Function2 ==
  data: Oy output; z input; Ox output
function [Oy, Ox]   = C3( z )
%C3 gives the rotation matrix about the z-axis for an angle 'z'
%   z - the angle about the z-axis which you rotate
%   A - the rotation matrix

Ox = [cos(z) sin(z); -sin(z) cos(z)]*[1;0];
Oy = [cos(z) sin(z); -sin(z) cos(z)]*[0;1];
end

== matlab function CLVF/Phase #2: Move to Initial Position/Change BLACK Behavior/Hough Control/MATLAB Function3 ==
  data: z input; Ox output
function Ox    = C3( z )
%C3 gives the rotation matrix about the z-axis for an angle 'z'
%   z - the angle about the z-axis which you rotate
%   A - the rotation matrix

Ox = [cos(z) sin(z); -sin(z) cos(z)]*[1;0];
end

== matlab function CLVF/Phase #2: Move to Initial Position/Change BLACK Behavior/Hough Control/MATLAB Function4 ==
  data: Oy input; e_out output; e_in input
function e_out = fcn(Oy, e_in)

a = sign(Oy'*e_in);
e_out = -a*norm(e_in);

== matlab function CLVF/From Force//Torque to PWM Signal/Change BLACK Behavior/Calculate Thruster ON//OFF/MATLAB Function ==
  data: H output; thruster_dist2CG_BLACK parameter; F_thrusters_BLACK parameter
function H = MakeH(thruster_dist2CG_BLACK,F_thrusters_BLACK)

Vec1 = [ -1
         -1
          0 
          0
          1
          1
          0
          0 ];
      
Vec2 = [  0
          0
          1
          1
          0
          0
         -1
         -1 ];
     
Vec3 = thruster_dist2CG_BLACK./1000;

Mat1 = [Vec1, Vec2, Vec3]';

Mat2 = diag((F_thrusters_BLACK./2));

H    = Mat1*Mat2;

end

== matlab function CLVF/Phase #3: Experiment/Change BLACK Behavior/Sub-Phase #4/BLACK_RzD/Wrap1/MATLAB Function ==
  data: u input; wrappedAngle output
function wrappedAngle = wrapAngle(u)

wrappedAngle = atan2(sin(u),cos(u));

end

== matlab function CLVF/Phase #3: Experiment/Change BLACK Behavior/Sub-Phase #4/Hough Control/MATLAB Function2 ==
  data: Oy output; z input; Ox output
function [Oy, Ox]   = C3( z )
%C3 gives the rotation matrix about the z-axis for an angle 'z'
%   z - the angle about the z-axis which you rotate
%   A - the rotation matrix

Ox = [cos(z) sin(z); -sin(z) cos(z)]*[1;0];
Oy = [cos(z) sin(z); -sin(z) cos(z)]*[0;1];
end

== matlab function CLVF/From Force//Torque to PWM Signal/Change BLACK Behavior/Calculate Thruster ON//OFF/MATLAB Function1 ==
  data: H output; thruster_dist2CG_BLACK parameter; F_thrusters_BLACK parameter
function H = MakeH(thruster_dist2CG_BLACK,F_thrusters_BLACK)

Vec1 = [ -1
         -1
          0 
          0
          1
          1
          0
          0 ];
      
Vec2 = [  0
          0
          1
          1
          0
          0
         -1
         -1 ];
     
Vec3 = thruster_dist2CG_BLACK./1000;

Mat1 = [Vec1, Vec2, Vec3]';

Mat2 = diag((F_thrusters_BLACK));

H    = Mat1*Mat2;

end

== matlab function CLVF/From Force//Torque to PWM Signal/Change BLACK Behavior/Calculate Thruster ON//OFF/MATLAB Function2 ==
  data: ThrustPer_Final output; ThrustPer input
function ThrustPer_Final  = ThrusterSat(ThrustPer)

ValveTime       = 0.007;
TControl        = 0.1;
ThrustPer_Final = zeros(8,1);

if max(ThrustPer) > 1
    ThrustPer_Sat = ThrustPer/max(ThrustPer);
else
    ThrustPer_Sat = ThrustPer;
end

for i = 1:8
    if ThrustPer_Sat(i) > ValveTime/TControl 
        ThrustPer_Final(i) = ThrustPer_Sat(i);
    else
        ThrustPer_Final(i) = 0;
    end
end
   

end

== matlab function CLVF/From Force//Torque to PWM Signal/Change BLACK Behavior/Calculate Thruster ON//OFF/Rotate Forces to Inertial/Create Rotation Matrix ==
  data: Rz input; C_Ib output
function C_Ib = RotateFrame(Rz)

C_bI = [  cos(Rz) sin(Rz)
         -sin(Rz) cos(Rz) ];

C_Ib = inv(C_bI);

end

== matlab function CLVF/From Force//Torque to PWM Signal/Change BLACK Behavior/Rotate Forces to Body/Create Rotation Matrix ==
  data: Rz input; C_bI output
function C_bI = RotateFrame(Rz)

C_bI = [  cos(Rz) sin(Rz)
         -sin(Rz) cos(Rz) ];

end

== matlab function CLVF/From Force//Torque to PWM Signal/Change RED Behavior/Calculate Thruster ON//OFF/MATLAB Function ==
  data: H output; thruster_dist2CG_RED parameter; F_thrusters_RED parameter
function H = MakeH(thruster_dist2CG_RED,F_thrusters_RED)

Vec1 = [ -1
         -1
          0 
          0
          1
          1
          0
          0 ];
      
Vec2 = [  0
          0
          1
          1
          0
          0
         -1
         -1 ];
     
Vec3 = thruster_dist2CG_RED./1000;

Mat1 = [Vec1, Vec2, Vec3]';

Mat2 = diag((F_thrusters_RED./2));

H    = Mat1*Mat2;

end

== matlab function CLVF/From Force//Torque to PWM Signal/Change RED Behavior/Calculate Thruster ON//OFF/MATLAB Function1 ==
  data: H output; thruster_dist2CG_RED parameter; F_thrusters_RED parameter
function H = MakeH(thruster_dist2CG_RED,F_thrusters_RED)

Vec1 = [ -1
         -1
          0 
          0
          1
          1
          0
          0 ];
      
Vec2 = [  0
          0
          1
          1
          0
          0
         -1
         -1 ];
     
Vec3 = thruster_dist2CG_RED./1000;

Mat1 = [Vec1, Vec2, Vec3]';

Mat2 = diag((F_thrusters_RED));

H    = Mat1*Mat2;

end

== matlab function CLVF/From Force//Torque to PWM Signal/Change RED Behavior/Calculate Thruster ON//OFF/MATLAB Function2 ==
  data: ThrustPer_Final output; ThrustPer input
function ThrustPer_Final  = ThrusterSat(ThrustPer)

ValveTime       = 0.007;
TControl        = 0.1;
ThrustPer_Final = zeros(8,1);

if max(ThrustPer) > 1
    ThrustPer_Sat = ThrustPer/max(ThrustPer);
else
    ThrustPer_Sat = ThrustPer;
end

for i = 1:8
    if ThrustPer_Sat(i) > ValveTime/TControl 
        ThrustPer_Final(i) = ThrustPer_Sat(i);
    else
        ThrustPer_Final(i) = 0;
    end
end
   

end

== matlab function CLVF/From Force//Torque to PWM Signal/Change RED Behavior/Calculate Thruster ON//OFF/Rotate Forces to Inertial/Create Rotation Matrix ==
  data: Rz input; C_Ib output
function C_Ib = RotateFrame(Rz)

C_bI = [  cos(Rz) sin(Rz)
         -sin(Rz) cos(Rz) ];

C_Ib = inv(C_bI);

end

== matlab function CLVF/Simulate Plant Dynamics/Sample and Hold Data to Match PhaseSpace (RED)/MATLAB Function ==
  data: TIME input; y output; SERVER input
function y = fcn(TIME, SERVER)

if mod(TIME,SERVER) == 0
    y = 1;
else
    y = 0;
end

== matlab function CLVF/Simulate Plant Dynamics/Sample and Hold Data to Match PhaseSpace (BLACK)/MATLAB Function ==
  data: TIME input; y output; SERVER input
function y = fcn(TIME, SERVER)

if mod(TIME,SERVER) == 0
    y = 1;
else
    y = 0;
end

== matlab function CLVF/From Force//Torque to PWM Signal/Change RED Behavior/Rotate Forces to Body/Create Rotation Matrix ==
  data: Rz input; C_bI output
function C_bI = RotateFrame(Rz)

C_bI = [  cos(Rz) sin(Rz)
         -sin(Rz) cos(Rz) ];

end

== matlab function CLVF/Phase #2: Move to Initial Position/Change RED Behavior/Hough Control/MATLAB Function2 ==
  data: Oy output; z input; Ox output
function [Oy, Ox]   = C3( z )
%C3 gives the rotation matrix about the z-axis for an angle 'z'
%   z - the angle about the z-axis which you rotate
%   A - the rotation matrix

Ox = [cos(z) sin(z); -sin(z) cos(z)]*[1;0];
Oy = [cos(z) sin(z); -sin(z) cos(z)]*[0;1];
end

== matlab function CLVF/Phase #2: Move to Initial Position/Change RED Behavior/Hough Control/MATLAB Function3 ==
  data: z input; Ox output
function Ox    = C3( z )
%C3 gives the rotation matrix about the z-axis for an angle 'z'
%   z - the angle about the z-axis which you rotate
%   A - the rotation matrix

Ox = [cos(z) sin(z); -sin(z) cos(z)]*[1;0];
end

== matlab function CLVF/Phase #2: Move to Initial Position/Change RED Behavior/Hough Control/MATLAB Function4 ==
  data: Oy input; e_out output; e_in input
function e_out = fcn(Oy, e_in)

a = sign(Oy'*e_in);
e_out = -a*norm(e_in);

== matlab function CLVF/Phase #3: Experiment/Change BLACK Behavior/Sub-Phase #4/Hough Control/MATLAB Function3 ==
  data: z input; Ox output
function Ox    = C3( z )
%C3 gives the rotation matrix about the z-axis for an angle 'z'
%   z - the angle about the z-axis which you rotate
%   A - the rotation matrix

Ox = [cos(z) sin(z); -sin(z) cos(z)]*[1;0];
end

== matlab function CLVF/Phase #4: Return Home/Change BLACK Behavior/Hough Control/MATLAB Function2 ==
  data: Oy output; z input; Ox output
function [Oy, Ox]   = C3( z )
%C3 gives the rotation matrix about the z-axis for an angle 'z'
%   z - the angle about the z-axis which you rotate
%   A - the rotation matrix

Ox = [cos(z) sin(z); -sin(z) cos(z)]*[1;0];
Oy = [cos(z) sin(z); -sin(z) cos(z)]*[0;1];
end

== matlab function CLVF/Phase #4: Return Home/Change BLACK Behavior/Hough Control/MATLAB Function3 ==
  data: z input; Ox output
function Ox    = C3( z )
%C3 gives the rotation matrix about the z-axis for an angle 'z'
%   z - the angle about the z-axis which you rotate
%   A - the rotation matrix

Ox = [cos(z) sin(z); -sin(z) cos(z)]*[1;0];
end

== matlab function CLVF/Phase #4: Return Home/Change BLACK Behavior/Hough Control/MATLAB Function4 ==
  data: Oy input; e_out output; e_in input
function e_out = fcn(Oy, e_in)

a = sign(Oy'*e_in);
e_out = -a*norm(e_in);

== matlab function CLVF/Phase #4: Return Home/Change RED Behavior/Hough Control/MATLAB Function2 ==
  data: Oy output; z input; Ox output
function [Oy, Ox]   = C3( z )
%C3 gives the rotation matrix about the z-axis for an angle 'z'
%   z - the angle about the z-axis which you rotate
%   A - the rotation matrix

Ox = [cos(z) sin(z); -sin(z) cos(z)]*[1;0];
Oy = [cos(z) sin(z); -sin(z) cos(z)]*[0;1];
end

== matlab function CLVF/Phase #4: Return Home/Change RED Behavior/Hough Control/MATLAB Function3 ==
  data: z input; Ox output
function Ox    = C3( z )
%C3 gives the rotation matrix about the z-axis for an angle 'z'
%   z - the angle about the z-axis which you rotate
%   A - the rotation matrix

Ox = [cos(z) sin(z); -sin(z) cos(z)]*[1;0];
end

== matlab function CLVF/Phase #4: Return Home/Change RED Behavior/Hough Control/MATLAB Function4 ==
  data: Oy input; e_out output; e_in input
function e_out = fcn(Oy, e_in)

a = sign(Oy'*e_in);
e_out = -a*norm(e_in);

== matlab function CLVF/Phase #2: Move to Initial Position/Change BLUE Behavior/Hough Control/MATLAB Function2 ==
  data: Oy output; z input; Ox output
function [Oy, Ox]   = C3( z )
%C3 gives the rotation matrix about the z-axis for an angle 'z'
%   z - the angle about the z-axis which you rotate
%   A - the rotation matrix

Ox = [cos(z) sin(z); -sin(z) cos(z)]*[1;0];
Oy = [cos(z) sin(z); -sin(z) cos(z)]*[0;1];
end

== matlab function CLVF/Phase #2: Move to Initial Position/Change BLUE Behavior/Hough Control/MATLAB Function3 ==
  data: z input; Ox output
function Ox    = C3( z )
%C3 gives the rotation matrix about the z-axis for an angle 'z'
%   z - the angle about the z-axis which you rotate
%   A - the rotation matrix

Ox = [cos(z) sin(z); -sin(z) cos(z)]*[1;0];
end

== matlab function CLVF/Phase #2: Move to Initial Position/Change BLUE Behavior/Hough Control/MATLAB Function4 ==
  data: Oy input; e_out output; e_in input
function e_out = fcn(Oy, e_in)

a = sign(Oy'*e_in);
e_out = -a*norm(e_in);

== matlab function CLVF/Phase #3: Experiment/Change BLACK Behavior/Sub-Phase #4/Lyapunov GNC/Navigation/getRotationMatrix ==
  data: u input; y output
function y = fcn(u)

y = C3(u);

== matlab function CLVF/Phase #3: Experiment/Change BLACK Behavior/Sub-Phase #4/States in Target-Fixed Frame/Norm ==
  data: rC_T input; r output; theta_T input; theta output; o_hat_B parameter
function [r, theta] = fcn(rC_T, theta_T, o_hat_B)

r = sqrt(sum(rC_T.^2));
r_hat = rC_T/r;
% Get the rotation matrix:
C_BI = C3(theta_T);

% Output the angle between the chaser and the desired position:
theta = acos(r_hat'*C_BI'*o_hat_B);

end
